simulink model "BlackBox_Model"  (R2020a)
settings: Solver=FixedStepAuto  StartTime=0.0  StopTime=sim_time  FixedStep=Ts  RelTol=1e-3  EnableMultiTasking=on
values from neighbouring files (symbols this model uses):
  step_amplitude = step_amplitude*10    (= 10)    [BlackBoxModel_sim.m]
  step_time = 1    [BlackBoxModel_sim.m]
  Ts = 1e-3    (= 0.001)    [BlackBoxModel_sim.m]
settings Model: Creator=Amodio  LastModifiedBy=Mara
settings DataIOCC: ReturnWorkspaceOutputs=off
settings OptimizationCC: LifeSpan=inf
settings DebuggingCC: SFUnexpectedBacktrackingDiag=warning  SFNoUnconditionalDefaultTransitionDiag=warning  ArithmeticOperatorsInVariantConditions=warning
settings SFSimCC: SimUseLocalCustomCode=off  CustomCodeUndefinedFunction=UseInterfaceOnly
settings RTWCC: RTWUseLocalCustomCode=off
settings CodeAppCC: StateflowObjectComments=on
settings GRTTargetCC: TargetLangStandard=C89/C90 (ANSI)
settings ConfigComp: CovMetricSettings=dw  CovHtmlReporting=on  CovSaveCumulativeToWorkspaceVar=on  CovSaveSingleToWorkspaceVar=on  CovExternalEMLEnable=off

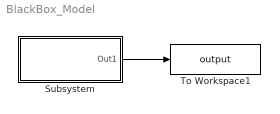
== system BlackBox_Model ==
  Subsystem : Subsystem
  To Workspace1 : ToWorkspace  VariableName=output  SampleTime=-1
  wires:
  Subsystem/1(Out1) -> To Workspace1/1

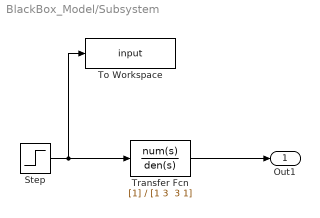
== system BlackBox_Model/Subsystem ==
  Step : Step  Time=step_time  After=step_amplitude  SampleTime=Ts
  To Workspace : ToWorkspace  VariableName=input  SampleTime=-1
  Transfer Fcn : TransferFcn  Denominator="[1 3  3 1]"
  Out1 : Outport
  wires:
  Step/1 -> Transfer Fcn/1, To Workspace/1
  Transfer Fcn/1 -> Out1/1
